simulink subsystem "pm_foc_decouple"  (R2022b)
settings: Solver=VariableStepAuto  StartTime=0.0  StopTime=10.0  RelTol=1e-3
settings Model: Creator=jack  LastModifiedBy=jack

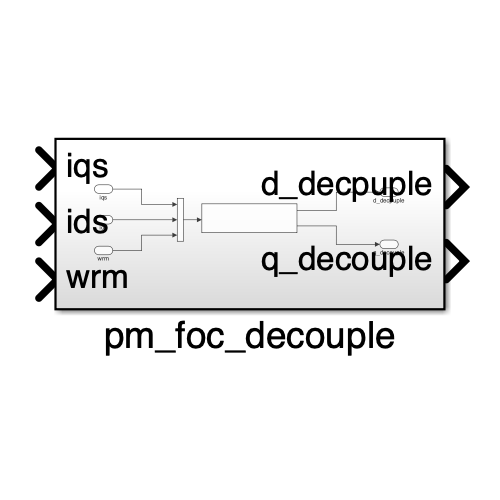
[thumbnail: Simulink's stored preview of the top-level diagram]
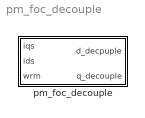
== system pm_foc_decouple ==
  pm_foc_decouple : Subsystem

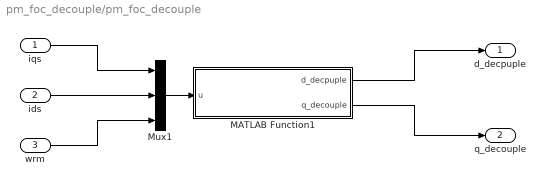
== system pm_foc_decouple/pm_foc_decouple ==
  iqs : Inport
  ids : Inport  Port=2
  wrm : Inport  Port=3
  MATLAB Function1 : MATLAB Function  TreatAsAtomicUnit=on
  Mux1 : Mux  Inputs=3
  d_decpuple : Outport
  q_decouple : Outport  Port=2
  wires:
  wrm/1 -> Mux1/3
  MATLAB Function1/2(q_decouple) -> q_decouple/1
  Mux1/1 -> MATLAB Function1/1(u)
  ids/1 -> Mux1/2
  MATLAB Function1/1(d_decpuple) -> d_decpuple/1
  iqs/1 -> Mux1/1

== matlab function pm_foc_decouple/MATLAB Function1 ==
  data: u input; d_decpuple output; q_decouple output
function [d_decpuple, q_decouple] = decouple(u)
    Ld = 0.0057;
    Lq = 0.0125;
    Lamda_f = 0.123;
    pole = 4;
    wr = u(3)*pole/2;
    d_decpuple = wr*(Lq/Ld)*u(1);
    q_decouple = wr*(Ld*u(2)+Lamda_f)/Lq;
